simulink model "GCS"  (R2026a)
settings: configuration reference "quad_config" (kept outside this file)
undefined symbols (not defined in the file): landTime, ts_comms
libraries: simulink x3
settings Model: DataDictionary=QuadData.sldd  ModifiedByFormat=The MathWorks, Inc.  Creator=The MathWorks, Inc.  LastModifiedBy=The MathWorks, Inc.
settings ConfigSetRef: SourceName=quad_config

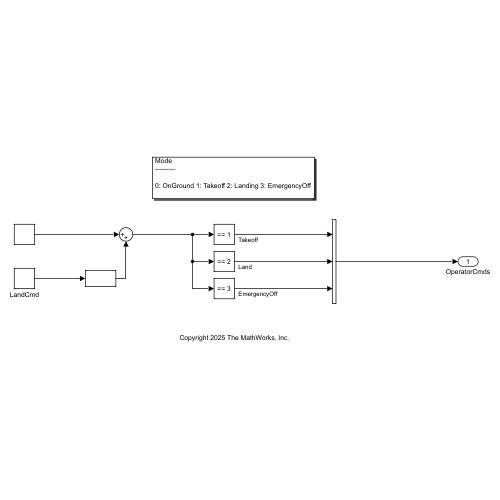
[thumbnail: Simulink's stored preview of the top-level diagram]
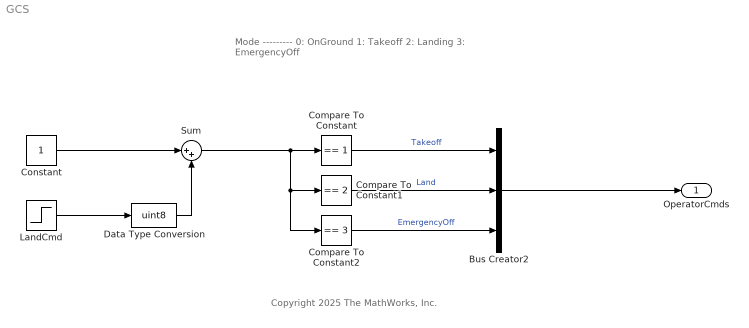
== system GCS ==
  note: Mode
      | ---------
      |
      | 0: OnGround 1: Takeoff 2: Landing 3: EmergencyOff
  note: Copyright 2025 The MathWorks, Inc.
  Bus Creator2 : BusCreator  Inputs=3  OutDataTypeStr=Bus: OperatorCmds  NonVirtualBus=on
  Compare To Constant : simulink/Logic and Bit Operations/Compare To Constant  relop===  const=1  OutDataTypeStr=boolean  ZeroCross=off
  Compare To Constant1 : simulink/Logic and Bit Operations/Compare To Constant  relop===  const=2  OutDataTypeStr=boolean  ZeroCross=off
  Compare To Constant2 : simulink/Logic and Bit Operations/Compare To Constant  relop===  const=3  OutDataTypeStr=boolean  ZeroCross=off
  Constant : Constant  OutDataTypeStr=uint8
  Data Type Conversion : DataTypeConversion  OutDataTypeStr=uint8  SaturateOnIntegerOverflow=off  RndMeth=Floor
  LandCmd : Step  Time=landTime  SampleTime=ts_comms
  Sum : Sum  Inputs=|++
  OperatorCmds : Outport  SampleTime=ts_comms  BusOutputAsStruct=on
  wires:
  LandCmd/1 -> Data Type Conversion/1
  Constant/1 -> Sum/1
  Data Type Conversion/1 -> Sum/2
  Sum/1 -> Compare To Constant2/1, Compare To Constant1/1, Compare To Constant/1
  Compare To Constant2/1 -> Bus Creator2/3  "EmergencyOff"
  Compare To Constant/1 -> Bus Creator2/1  "Takeoff"
  Bus Creator2/1 -> OperatorCmds/1
  Compare To Constant1/1 -> Bus Creator2/2  "Land"
